simulink model "project2"  (R2024a)
settings: Solver=VariableStepAuto  StartTime=0.0  StopTime=10.0  RelTol=1e-3
libraries: simulink x1
settings Model: Creator=robin  LastModifiedBy=robin

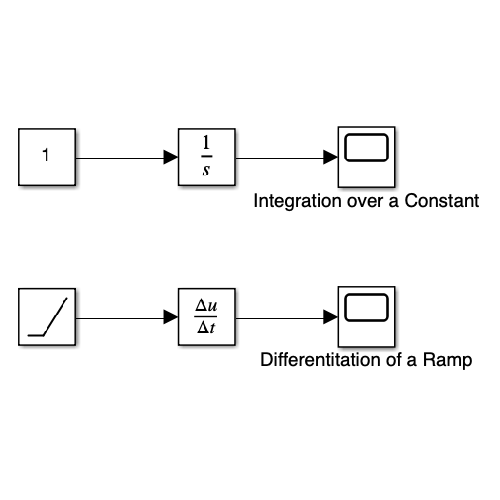
[thumbnail: Simulink's stored preview of the top-level diagram]
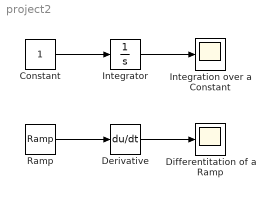
== system project2 ==
  Constant : Constant
  Derivative : Derivative
  Differentitation of a Ramp : Scope
  Integration over a Constant : Scope
  Integrator : Integrator
  Ramp : simulink/Sources/Ramp  slope=1  start=0  InitialOutput=0
  wires:
  Constant/1 -> Integrator/1
  Integrator/1 -> Integration over a Constant/1
  Derivative/1 -> Differentitation of a Ramp/1
  Ramp/1 -> Derivative/1
